simulink model "eg4"  (R2015a)
settings: Solver=ode45  StartTime=0.0  StopTime=150  RelTol=1e-3
settings Model: Creator=Ayush Kumar Shah  LastModifiedBy=ayush

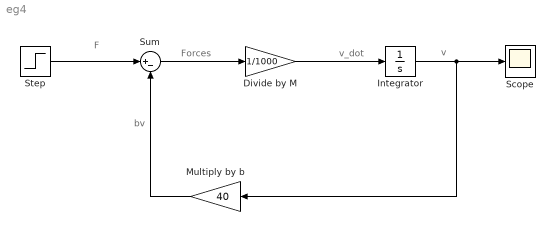
== system eg4 ==
  note: bv
  note: v
  note: v_dot
  note: Forces
  note: F
  Divide by M : Gain  Gain=1/1000
  Integrator : Integrator
  Multiply by b : Gain  Gain=40
  Scope : Scope
  Step : Step  Time=0  After=400  SampleTime=0
  Sum : Sum  Inputs=|+-
  wires:
  Sum/1 -> Divide by M/1
  Divide by M/1 -> Integrator/1
  Integrator/1 -> Multiply by b/1, Scope/1
  Step/1 -> Sum/1
  Multiply by b/1 -> Sum/2
